simulink model "tethersMoment_th"  (R2018b)
settings: Solver=VariableStepAuto  StartTime=0.0  StopTime=0  RelTol=1e-3
values from neighbouring files (symbols this model uses):
  frc1 = [1 0 0]    [tethersMoment_ts.m]
  frc2 = [1 0 0]    [tethersMoment_ts.m]
  frc3 = [-1 0 0]    [tethersMoment_ts.m]
  rotMat = eye(3)    [tethersMoment_ts.m]
undefined symbols (not defined in the file or in its folder): arms
libraries: tethersMoment_cl x1
settings Model: Creator=mcobb  LastModifiedBy=mcobb

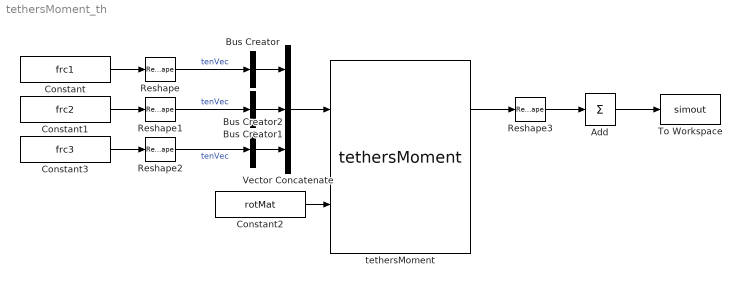
== system tethersMoment_th ==
  Add : Sum  Inputs=+  CollapseMode=Specified dimension  CollapseDim=2
  Bus Creator : BusCreator  Inputs=1  OutDataTypeStr=Bus: singleBus  NonVirtualBus=on
  Bus Creator1 : BusCreator  Inputs=1  OutDataTypeStr=Bus: singleBus  NonVirtualBus=on
  Bus Creator2 : BusCreator  Inputs=1  OutDataTypeStr=Bus: singleBus  NonVirtualBus=on
  Constant : Constant  Value=frc1
  Constant1 : Constant  Value=frc2
  Constant2 : Constant  Value=rotMat
  Constant3 : Constant  Value=frc3
  Reshape : Reshape  OutputDimensionality=Column vector (2-D)
  Reshape1 : Reshape  OutputDimensionality=Column vector (2-D)
  Reshape2 : Reshape  OutputDimensionality=Column vector (2-D)
  Reshape3 : Reshape  OutputDimensionality=Customize  OutputDimensions=[3 numel(arms)]
  To Workspace : ToWorkspace  VariableName=simout  SaveFormat=Timeseries  SampleTime=-1
  Vector Concatenate : Concatenate  NumInputs=3
  tethersMoment : tethersMoment_cl/tethersMoment  arms=arms
  wires:
  Bus Creator/1 -> Vector Concatenate/1
  Constant/1 -> Reshape/1
  Constant1/1 -> Reshape1/1
  Constant2/1 -> tethersMoment/2
  tethersMoment/1 -> Reshape3/1
  Constant3/1 -> Reshape2/1
  Reshape/1 -> Bus Creator/1  "tenVec"
  Reshape1/1 -> Bus Creator1/1  "tenVec"
  Reshape2/1 -> Bus Creator2/1  "tenVec"
  Bus Creator1/1 -> Vector Concatenate/2
  Bus Creator2/1 -> Vector Concatenate/3
  Vector Concatenate/1 -> tethersMoment/1
  Reshape3/1 -> Add/1
  Add/1 -> To Workspace/1
